simulink model "Merged_Simulink_Modes_FinalV2"  (R2020a)
settings: Solver=FixedStepAuto  StartTime=0.0  StopTime=10.0  FixedStep=1e-3  RelTol=1e-3  EnableMultiTasking=on
undefined symbols (not defined in the file): D0, D1, D10, D11, D12, D13, D2, D3, D4, D5, D6, D7, D8, D9, PTA0, PTA1, PTA2, PTB23, PTB9, PTC16, PTC17, PTC2, PTC3, PTC4, PTD0, PTD1, PTD2, PTD3
libraries: frdmk64flib x19, dspstat3 x1
settings Model: ExtModeTrigDuration=5  Creator=karir  LastModifiedBy=guga
settings OptimizationCC: EnhancedBackFolding=on  PassReuseOutputArgsAs=Individual arguments  ZeroExternalMemoryAtStartup=off  ZeroInternalMemoryAtStartup=off  MaxStackSize=64  OptimizeBlockOrder=speed  DifferentSizesBufferReuse=on  OptimizationCustomize=off  EfficientTunableParamExpr=on
settings DebuggingCC: ParameterTunabilityLossMsg=error
settings HardwareCC: ProdBitPerPointer=32  ProdBitPerSizeT=32  ProdBitPerPtrDiffT=32  ProdLargestAtomicInteger=Long  ProdLargestAtomicFloat=Double  ProdWordSize=32  ProdHWDeviceType=ARM Compatible->ARM Cortex
settings SFSimCC: MATLABDynamicMemAlloc=off
settings RTWCC: SystemTargetFile=ert.tlc  HardwareBoard=NXP FRDM-K64F  TemplateMakefile=ert_default_tmf  Toolchain=GNU Tools for ARM Embedded Processors
settings CodeAppCC: ForceParamTrailComments=on  IgnoreCustomStorageClasses=off  OperatorAnnotations=on  SimulinkDataObjDesc=on  SFDataObjDesc=on  InsertBlockDesc=on

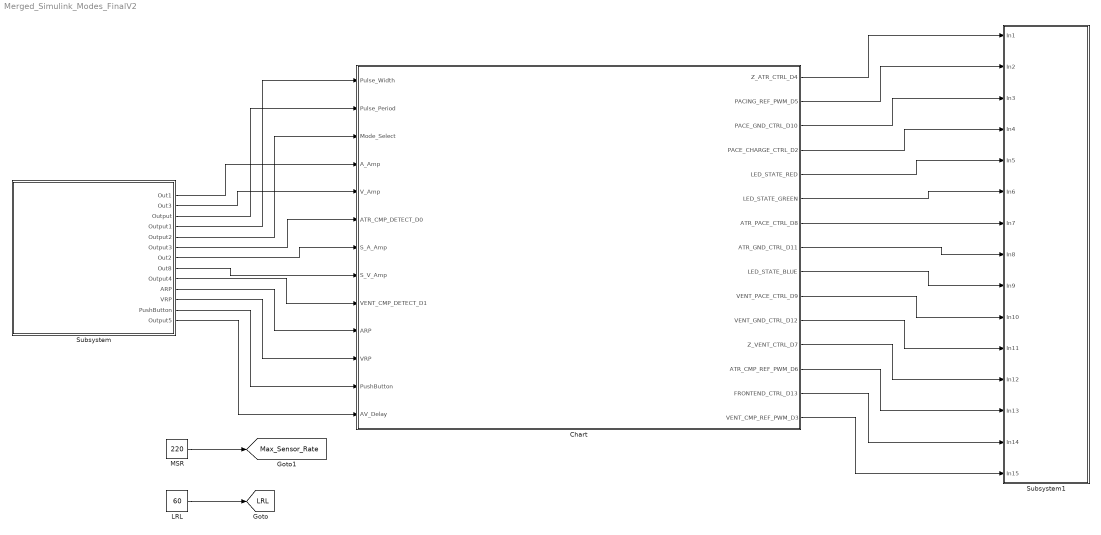
== system Merged_Simulink_Modes_FinalV2 ==
  Chart : Stateflow chart  TreatAsAtomicUnit=on
  LRL : Constant  Value=60  OutMin=30  OutMax=180  OutDataTypeStr=uint16
  MSR : Constant  Value=220  OutDataTypeStr=uint16
  Subsystem : Subsystem
  Subsystem1 : Subsystem
  tag scope: LRL=global, Max_Sensor_Rate=global
  wires:
  Subsystem/1(Out1) -> Chart/4(A_Amp)
  Subsystem/3(Output) -> Chart/2(Pulse_Period)
  Subsystem/4(Output1) -> Chart/1(Pulse_Width)
  Subsystem/5(Output2) -> Chart/3(Mode_Select)
  Chart/1(Z_ATR_CTRL_D4) -> Subsystem1/1(In1)
  Chart/2(PACING_REF_PWM_D5) -> Subsystem1/2(In2)
  Chart/3(PACE_GND_CTRL_D10) -> Subsystem1/3(In3)
  Chart/4(PACE_CHARGE_CTRL_D2) -> Subsystem1/4(In4)
  Chart/5(LED_STATE_RED) -> Subsystem1/5(In5)
  Chart/6(LED_STATE_GREEN) -> Subsystem1/6(In6)
  Chart/7(ATR_PACE_CTRL_D8) -> Subsystem1/7(In7)
  Chart/8(ATR_GND_CTRL_D11) -> Subsystem1/8(In8)
  Chart/9(LED_STATE_BLUE) -> Subsystem1/9(In9)
  Chart/10(VENT_PACE_CTRL_D9) -> Subsystem1/10(In10)
  Chart/11(VENT_GND_CTRL_D12) -> Subsystem1/11(In11)
  Chart/12(Z_VENT_CTRL_D7) -> Subsystem1/12(In12)
  Subsystem/6(Output3) -> Chart/6(ATR_CMP_DETECT_D0)
  Subsystem/7(Out2) -> Chart/7(S_A_Amp)
  Chart/13(ATR_CMP_REF_PWM_D6) -> Subsystem1/13(In13)
  Chart/14(FRONTEND_CTRL_D13) -> Subsystem1/14(In14)
  Subsystem/9(Output4) -> Chart/9(VENT_CMP_DETECT_D1)
  Chart/15(VENT_CMP_REF_PWM_D3) -> Subsystem1/15(In15)
  Subsystem/11(VRP) -> Chart/11(VRP)
  Subsystem/12(PushButton) -> Chart/12(PushButton)
  Subsystem/10(ARP) -> Chart/10(ARP)
  LRL/1 -> [LRL]
  MSR/1 -> [Max_Sensor_Rate]
  Subsystem/13(Output5) -> Chart/13(AV_Delay)
  Subsystem/2(Out3) -> Chart/5(V_Amp)
  Subsystem/8(Out8) -> Chart/8(S_V_Amp)

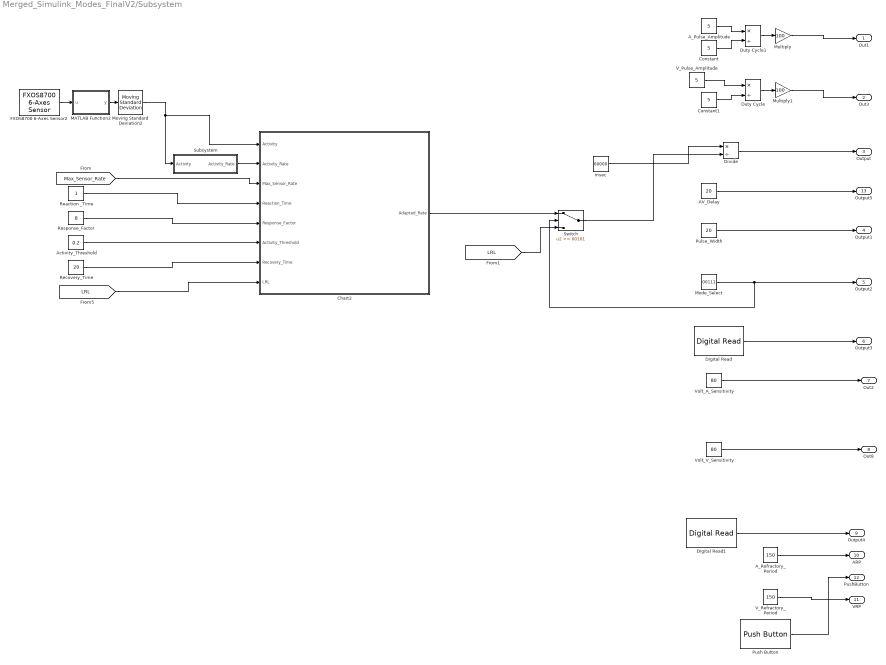
== system Merged_Simulink_Modes_FinalV2/Subsystem ==
  AV_Delay : Constant  Value=20  OutMin=[0]  OutMax=20  OutDataTypeStr=uint16  LockScale=on
  A_Pulse_Amplitude : Constant  Value=5
  A_Refractory_Period : Constant  Value=150
  Activity_Threshold : Constant  Value=0.2  OutDataTypeStr=double
  Chart2 : Stateflow chart  TreatAsAtomicUnit=on
  Constant : Constant  Value=5
  Constant1 : Constant  Value=5
  Digital Read : frdmk64flib/Digital Read  Whichpin=PTC16 (D0)  SampleTime=-1
  Digital Read1 : frdmk64flib/Digital Read  Whichpin=PTC17 (D1)  SampleTime=-1
  Divide : Product  Inputs=*/
  Duty Cycle : Product  Inputs=*/
  Duty Cycle1 : Product  Inputs=*/
  FXOS8700 6-Axes Sensor2 : frdmk64flib/FXOS8700 6-Axes Sensor  Activesensor=Accelerometer only  ODR=100Hz  HybridODR=400Hz  Accelfullrange=-4g to +4g  SampleTime=1/100
  MATLAB Function2 : MATLAB Function  TreatAsAtomicUnit=on
  Mode_Select : Constant  Value=00111
  Moving Standard Deviation2 : dspstat3/Moving Standard Deviation  Method=Sliding window  ForgettingFactorPort=off  SpecifyWindowLength=on  WindowLength=100  ForgettingFactor=0.9  SimulateUsing=Code generation
      settings: SourceProductBaseCode=DS
  Multiply : Gain  Gain=100
  Multiply1 : Gain  Gain=100
  Pulse_Width : Constant  Value=20  OutMin=[0]  OutMax=20  OutDataTypeStr=uint16  LockScale=on
  Push Button : frdmk64flib/Push Button  Whichswitch=SW2  SampleTime1=-1
  "Reaction\t_Time " : Constant  OutDataTypeStr=uint16
  Recovery_Time : Constant  Value=20  OutDataTypeStr=uint16
  Response_Factor : Constant  Value=8  OutDataTypeStr=double  LockScale=on
  Subsystem : Subsystem
  Switch : Switch  Threshold=00101
  V_Pulse_Amplitude : Constant  Value=5
  V_Refractory_Period : Constant  Value=150
  Volt_A_Sensitivity : Constant  Value=80
  Volt_V_Sensitivity : Constant  Value=80
  msec : Constant  Value=60000
  Out1 : Outport
  Out3 : Outport  Port=2
  Output : Outport  Port=3
  Output1 : Outport  Port=4
  Output2 : Outport  Port=5
  Output3 : Outport  Port=6
  Out2 : Outport  Port=7
  Out8 : Outport  Port=8
  Output4 : Outport  Port=9
  ARP : Outport  Port=10
  VRP : Outport  Port=11
  PushButton : Outport  Port=12
  Output5 : Outport  Port=13
  wires:
  msec/1 -> Divide/1
  Pulse_Width/1 -> Output1/1
  Divide/1 -> Output/1
  Digital Read/1 -> Output3/1
  Volt_A_Sensitivity/1 -> Out2/1
  Digital Read1/1 -> Output4/1
  A_Refractory_Period/1 -> ARP/1
  V_Refractory_Period/1 -> VRP/1
  Push Button/1 -> PushButton/1
  FXOS8700 6-Axes Sensor2/1 -> MATLAB Function2/1(u)
  [LRL] -> Switch/3
  Recovery_Time/1 -> Chart2/7(Recovery_Time)
  MATLAB Function2/1(y) -> Moving Standard Deviation2/1
  [LRL] -> Chart2/8(LRL)
  Moving Standard Deviation2/1 -> Chart2/1(Activity), Subsystem/1(Activity)
  Activity_Threshold/1 -> Chart2/6(Activity_Threshold)
  Subsystem/1(Activity_Rate) -> Chart2/2(Activity_Rate)
  Chart2/1(Adapted_Rate) -> Switch/1
  [Max_Sensor_Rate] -> Chart2/3(Max_Sensor_Rate)
  "Reaction\t_Time "/1 -> Chart2/4(Reaction_Time)
  Response_Factor/1 -> Chart2/5(Response_Factor)
  Mode_Select/1 -> Switch/2, Output2/1
  Switch/1 -> Divide/2
  AV_Delay/1 -> Output5/1
  V_Pulse_Amplitude/1 -> Duty Cycle/1
  Constant/1 -> Duty Cycle1/2
  Multiply/1 -> Out1/1
  A_Pulse_Amplitude/1 -> Duty Cycle1/1
  Multiply1/1 -> Out3/1
  Constant1/1 -> Duty Cycle/2
  Duty Cycle/1 -> Multiply1/1
  Duty Cycle1/1 -> Multiply/1
  Volt_V_Sensitivity/1 -> Out8/1

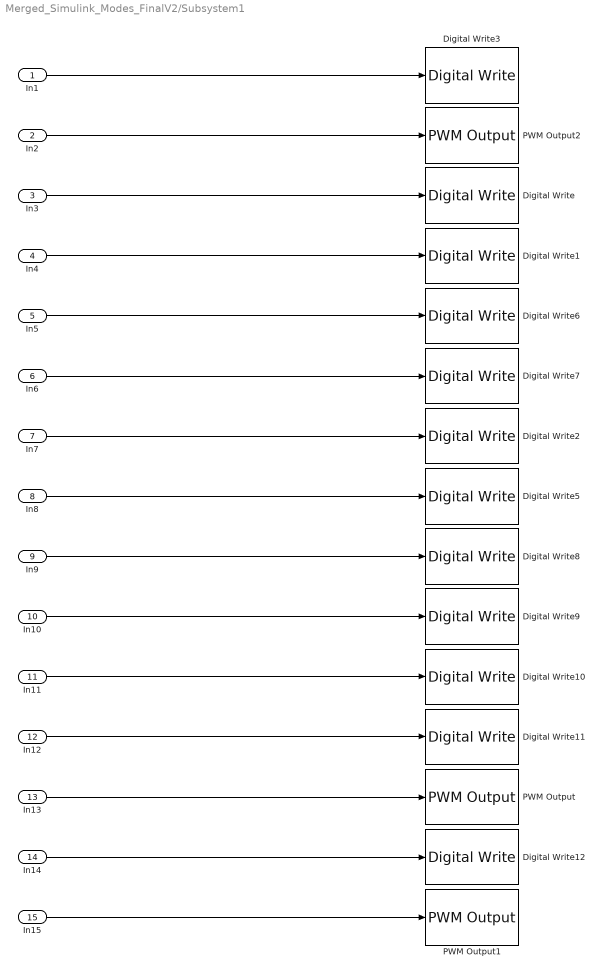
== system Merged_Simulink_Modes_FinalV2/Subsystem1 ==
  In1 : Inport
  In2 : Inport  Port=2
  In3 : Inport  Port=3
  In4 : Inport  Port=4
  In5 : Inport  Port=5
  In6 : Inport  Port=6
  In7 : Inport  Port=7
  In8 : Inport  Port=8
  In9 : Inport  Port=9
  In10 : Inport  Port=10
  In11 : Inport  Port=11
  In12 : Inport  Port=12
  In13 : Inport  Port=13
  In14 : Inport  Port=14
  In15 : Inport  Port=15
  Digital Write : frdmk64flib/Digital Write  Whichpin=PTD0 (D10)
  Digital Write1 : frdmk64flib/Digital Write  Whichpin=PTB9 (D2)
  Digital Write10 : frdmk64flib/Digital Write  Whichpin=PTD3 (D12)
  Digital Write11 : frdmk64flib/Digital Write  Whichpin=PTC3 (D7)
  Digital Write12 : frdmk64flib/Digital Write  Whichpin=PTD1 (D13)
  Digital Write2 : frdmk64flib/Digital Write  Whichpin=PTA0 (D8)
  Digital Write3 : frdmk64flib/Digital Write  Whichpin=PTB23 (D4)
  Digital Write5 : frdmk64flib/Digital Write  Whichpin=PTD2 (D11)
  Digital Write6 : frdmk64flib/Digital Write  Whichpin=RED_LED
  Digital Write7 : frdmk64flib/Digital Write  Whichpin=GREEN_LED
  Digital Write8 : frdmk64flib/Digital Write  Whichpin=BLUE_LED
  Digital Write9 : frdmk64flib/Digital Write  Whichpin=PTC4 (D9)
  PWM Output : frdmk64flib/PWM Output  Whichpin=PTC2 (D6)  InitialFrequency=2000  InitialDutyCycle=0
  PWM Output1 : frdmk64flib/PWM Output  Whichpin=PTA1 (D3)  InitialFrequency=2000  InitialDutyCycle=0
  PWM Output2 : frdmk64flib/PWM Output  Whichpin=PTA2 (D5)  InitialFrequency=2000  InitialDutyCycle=0
  wires:
  In6/1 -> Digital Write7/1
  In5/1 -> Digital Write6/1
  In1/1 -> Digital Write3/1
  In2/1 -> PWM Output2/1
  In4/1 -> Digital Write1/1
  In8/1 -> Digital Write5/1
  In7/1 -> Digital Write2/1
  In3/1 -> Digital Write/1
  In12/1 -> Digital Write11/1
  In9/1 -> Digital Write8/1
  In10/1 -> Digital Write9/1
  In11/1 -> Digital Write10/1
  In13/1 -> PWM Output/1
  In14/1 -> Digital Write12/1
  In15/1 -> PWM Output1/1

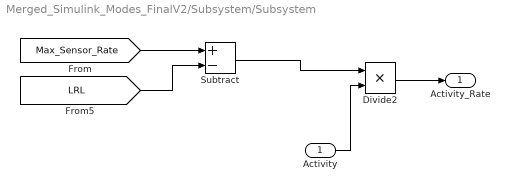
== system Merged_Simulink_Modes_FinalV2/Subsystem/Subsystem ==
  Activity : Inport
  Divide2 : Product  Inputs=**  OutDataTypeStr=uint16
  Subtract : Sum  Inputs=+-
  Activity_Rate : Outport  VectorParamsAs1DForOutWhenUnconnected=off
  wires:
  [Max_Sensor_Rate] -> Subtract/1
  [LRL] -> Subtract/2
  Subtract/1 -> Divide2/1
  Activity/1 -> Divide2/2
  Divide2/1 -> Activity_Rate/1

== stateflow chart Merged_Simulink_Modes_FinalV2/Chart ==
  state VOO
    state Charging
      entry:
      PACING_REF_PWM_D5 = V_Amp;
      PACE_CHARGE_CTRL_D2 = 1;
      VENT_PACE_CTRL_D9 = 0;
      VENT_GND_CTRL_D12 = 1;
      PACE_GND_CTRL_D10 = 0;
      Z_VENT_CTRL_D7 = 0;
      LED_STATE_RED = false;
      LED_STATE_BLUE = true;
    state Pacing
      entry:
      PACING_REF_PWM_D5 = V_Amp;
      PACE_CHARGE_CTRL_D2 = 0;
      VENT_PACE_CTRL_D9 = 1;
      VENT_GND_CTRL_D12 = 0;
      PACE_GND_CTRL_D10 = 1;
      Z_VENT_CTRL_D7 = 0;
      LED_STATE_RED = true;
      LED_STATE_BLUE = false;
    (default) -> Charging
    Charging -> VOO.Pacing : [after(Pulse_Period - Pulse_Width,msec)]
    VOO.Pacing -> Charging : [after(Pulse_Width,msec)]
  state AOO
    state Chambers_Paced_Charging
      entry:
      PACING_REF_PWM_D5 = A_Amp;
      PACE_CHARGE_CTRL_D2=1;
      ATR_PACE_CTRL_D8= 0;
      ATR_GND_CTRL_D11= 1;
      PACE_GND_CTRL_D10=0;
      Z_ATR_CTRL_D4=0;
      LED_STATE_RED=true;
      LED_STATE_GREEN=false;
    state pacing
      entry:
      PACING_REF_PWM_D5 = A_Amp;
      PACE_CHARGE_CTRL_D2=0;
      ATR_PACE_CTRL_D8= 1;
      ATR_GND_CTRL_D11= 0;
      PACE_GND_CTRL_D10=1;
      Z_ATR_CTRL_D4=0;
      LED_STATE_RED=false;
      LED_STATE_GREEN=true;
    (default) -> Chambers_Paced_Charging
    Chambers_Paced_Charging -> pacing : [after(Pulse_Period-Pulse_Width,msec)]
    pacing -> Chambers_Paced_Charging : [after(Pulse_Width,msec)]
  state VVI
    state Pacing1
      entry:
      PACING_REF_PWM_D5 = V_Amp;
      PACE_CHARGE_CTRL_D2 = 0;
      VENT_PACE_CTRL_D9 = 1;
      VENT_GND_CTRL_D12 = 0;
      PACE_GND_CTRL_D10 = 1;
      Z_VENT_CTRL_D7 = 0;
      LED_STATE_RED = true;
      LED_STATE_BLUE = false;
    state Charging_and_Sensing1
      entry:
      PACING_REF_PWM_D5 = V_Amp;
      PACE_CHARGE_CTRL_D2 = 1;
      VENT_PACE_CTRL_D9 = 0;
      VENT_GND_CTRL_D12 = 1;
      PACE_GND_CTRL_D10 = 0;
      Z_VENT_CTRL_D7 = 0;
      LED_STATE_RED = false;
      LED_STATE_BLUE = true;
      FRONTEND_CTRL_D13 = 1;
      VENT_CMP_REF_PWM_D3 = S_V_Amp;
    (default) -> Charging_and_Sensing1
    Pacing1 -> Charging_and_Sensing1 : [after(Pulse_Width,msec)]
    Charging_and_Sensing1 -> (junction 80) : after(VRP-Pulse_Width,msec)
    (junction 80) -> Pacing1 [order 2] : after(Pulse_Period-VRP,msec)[VENT_CMP_DETECT_D1 == 0 & PushButton == false]
    (junction 80) -> Charging_and_Sensing1 [order 1] : [VENT_CMP_DETECT_D1 == 1 | PushButton == true]
  state Start_State
  state AAI
    state Pacing
      entry:
      PACING_REF_PWM_D5 = A_Amp;
      PACE_CHARGE_CTRL_D2=0;
      ATR_PACE_CTRL_D8= 1;
      ATR_GND_CTRL_D11= 0;
      PACE_GND_CTRL_D10=1;
      Z_ATR_CTRL_D4=0;
      LED_STATE_RED=false;
      LED_STATE_GREEN=true;
    state Charging_and_Sensing
      entry:
      PACING_REF_PWM_D5 = A_Amp;
      PACE_CHARGE_CTRL_D2=1;
      ATR_PACE_CTRL_D8= 0;
      ATR_GND_CTRL_D11= 1;
      PACE_GND_CTRL_D10=0;
      Z_ATR_CTRL_D4=0;
      LED_STATE_RED=true;
      LED_STATE_GREEN=false;
      FRONTEND_CTRL_D13 = 1;
      ATR_CMP_REF_PWM_D6 = S_A_Amp;
    (default) -> Charging_and_Sensing
    AAI.Pacing -> Charging_and_Sensing : after(Pulse_Width,msec)
    Charging_and_Sensing -> (junction 90) : after(ARP-Pulse_Width, msec)
    (junction 90) -> AAI.Pacing [order 2] : after(Pulse_Period-ARP,msec)[ATR_CMP_DETECT_D0 == 0 & PushButton == false]
    (junction 90) -> Charging_and_Sensing [order 1] : [ATR_CMP_DETECT_D0 == 1 | PushButton == true]
  state DOO
    state AOO_Charging
      entry:
      LED_STATE_RED=true;
      LED_STATE_GREEN=false;
      LED_STATE_BLUE = false;
      PACING_REF_PWM_D5 = A_Amp;
      PACE_CHARGE_CTRL_D2=1;
      ATR_PACE_CTRL_D8= 0;
      ATR_GND_CTRL_D11= 1;
      PACE_GND_CTRL_D10=0;
      Z_ATR_CTRL_D4=0;
    state VOO_Charging
      entry:
      LED_STATE_RED=true;
      LED_STATE_GREEN=false;
      LED_STATE_BLUE = false;
      PACING_REF_PWM_D5 = V_Amp;
      PACE_CHARGE_CTRL_D2 = 1;
      VENT_PACE_CTRL_D9 = 0;
      VENT_GND_CTRL_D12 = 1;
      PACE_GND_CTRL_D10 = 0;
      Z_VENT_CTRL_D7 = 0;
    state VOO
      entry:
      PACING_REF_PWM_D5 = V_Amp;
      PACE_CHARGE_CTRL_D2 = 0;
      VENT_PACE_CTRL_D9 = 1;
      VENT_GND_CTRL_D12 = 0;
      PACE_GND_CTRL_D10 = 1;
      Z_VENT_CTRL_D7 = 0;
      LED_STATE_RED=false;
      LED_STATE_GREEN=false;
      LED_STATE_BLUE = true;
    state AOO
      entry:
      PACING_REF_PWM_D5 = A_Amp;
      PACE_CHARGE_CTRL_D2=0;
      ATR_PACE_CTRL_D8= 1;
      ATR_GND_CTRL_D11= 0;
      PACE_GND_CTRL_D10=1;
      Z_ATR_CTRL_D4=0;
      LED_STATE_RED=false;
      LED_STATE_GREEN=true;
      LED_STATE_BLUE = false;
    (default) -> AOO_Charging
    AOO_Charging -> DOO.AOO : [after(Pulse_Period-Pulse_Width,msec)]
    DOO.AOO -> VOO_Charging : [after(Pulse_Width,msec)]
    VOO_Charging -> DOO.VOO : [after(AV_Delay,msec)]
    DOO.VOO -> AOO_Charging : [after(2*Pulse_Width-AV_Delay,msec)]
  Start_State -> VOO [order 2] : [Mode_Select == 00001 | Mode_Select == 00110]
  VOO -> Start_State : [Mode_Select ~= 00001 & Mode_Select ~= 00110]
  (default) -> Start_State
  VVI -> Start_State : [Mode_Select ~= 00011 & Mode_Select ~= 01000]
  AOO -> Start_State : [Mode_Select ~= 00000 & Mode_Select ~= 00101]
  Start_State -> VVI [order 4] : [Mode_Select == 00011 | Mode_Select == 01000]
  Start_State -> AOO [order 1] : [Mode_Select == 00000 | Mode_Select == 00101]
  Start_State -> DOO [order 5] : [Mode_Select == 00100 | Mode_Select == 01001]
  AAI -> Start_State : [Mode_Select ~= 00010 & Mode_Select ~= 00111]
  Start_State -> AAI [order 3] : [Mode_Select == 00010 | Mode_Select == 00111]
  DOO -> Start_State : [Mode_Select ~= 00100 & Mode_Select ~= 01001]
  data: Z_ATR_CTRL_D4 output; PACING_REF_PWM_D5 output; PACE_GND_CTRL_D10 output; PACE_CHARGE_CTRL_D2 output; LED_STATE_RED output; LED_STATE_GREEN output; ATR_PACE_CTRL_D8 output; ATR_GND_CTRL_D11 output; Pulse_Width input; Pulse_Period input; Mode_Select input; A_Amp input; V_Amp input; LED_STATE_BLUE output; VENT_PACE_CTRL_D9 output; VENT_GND_CTRL_D12 output; Z_VENT_CTRL_D7 output; ATR_CMP_REF_PWM_D6 output; ATR_CMP_DETECT_D0 input; S_A_Amp input; S_V_Amp input; FRONTEND_CTRL_D13 output; VENT_CMP_DETECT_D1 input; ARP input; VENT_CMP_REF_PWM_D3 output; VRP input; PushButton input; AV_Delay input

== stateflow chart Merged_Simulink_Modes_FinalV2/Subsystem/Chart2 ==
  state Activity_Rate
  state Up
    entry:
    Time = 0;
    during:
    Adapted_Rate = Response_Factor*(Time/Reaction_Time)/(1+(Time/Reaction_Time)*(Response_Factor-1))*Activity_Rate + LRL;
    Time = Time + 1/1000;
    exit:
    Time = 0;
  state Max
    entry:
    Adapted_Rate = Max_Sensor_Rate;
  state Down
    entry:
    Time = 0;
    Rate_Diff = Adapted_Rate - LRL;
    during:
    Adapted_Rate = Adapted_Rate - (Rate_Diff/Recovery_Time)*Time;
    Time = Time + 1/1000;
    exit:
    Time = 0;
  state Start
    entry:
    Adapted_Rate = LRL;
  state Min
  Up -> Activity_Rate [order 2] : [Adapted_Rate>=Activity_Rate+LRL]
  Up -> Up [order 3] : [Time >= Reaction_Time]{Time = 0}
  Activity_Rate -> Down [order 2] : [Activity < Activity_Threshold]
  Activity_Rate -> Up [order 1] : [Activity >= Activity_Threshold]
  Up -> Max [order 1] : [Adapted_Rate >= Max_Sensor_Rate]
  Min -> Up : [Activity >= Activity_Threshold]
  Max -> Down : [Activity < Activity_Threshold]
  Up -> Down [order 4] : [Activity < Activity_Threshold]
  Down -> Up [order 1] : [Activity >= Activity_Threshold]
  (default) -> Start
  Start -> Down
  Down -> Min [order 2] : [Adapted_Rate == LRL]
  Down -> Down [order 3] : [Time >= Recovery_Time]{Time = 0}
  data: Activity input double; Activity_Rate input; Adapted_Rate output uint16; Max_Sensor_Rate input uint16; Reaction_Time input uint16; Response_Factor input double; Activity_Threshold input double; Recovery_Time input uint16; LRL input uint16; Rate_Diff local uint16; Time local double

== matlab function Merged_Simulink_Modes_FinalV2/Subsystem/MATLAB Function2 ==
  data: u input; y output
function y = fcn(u)
y = sqrt(u(1)^2+u(2)^2+u(3)^2);
